simulink model "pumaModel"  (R2021b)
settings: Solver=VariableStepAuto  StartTime=0.0  StopTime=stopTime  FixedStep=.0001  RelTol=1e-3
values from neighbouring files (symbols this model uses):
  C = [0 c12_1*dq1 c13_1*dq3;c11_2*dq1 0 c22_2*dq2+c23_2*dq3;c11_3*dq1 c22_3*dq2 0]    [puma560ModifiedDynamics.m]
  dq_0 = [0 0 0]    [matlab.mat]
  fdControl = 2    [InitializationScript.m]
  fEE = 0    [InitializationScript.m]    (also in matlab.mat = 100)
  IC = [0;0;0]    [InitializationScript.m]    (also in matlab.mat = [0 0 0])
  m = 3    [matlab.mat]
  pathPoints = [IC,solution1,solution2,solution3,solution4,solution5,solution6]    [InitializationScript.m]    (also in matlab.mat = [0 0 0 4.71238898038 -1.57079632679 3.14159265359 3.14159265)
  q_0 = [0 0 0]    [matlab.mat]
  timePoints = [0 2 4 6 8 10 12]    [InitializationScript.m]    (also in matlab.mat = [0 2 4 6 8])
  velPoints = zeros(3,7)    [InitializationScript.m]    (also in matlab.mat = [0 0 0 0 0 0 0 0 0 0 0 0 ... (15 elements, 3x5)])
  X = [cos(q1)*(l2*cos(q2)+l3*sin(q2+q3));sin(q1)*(l2*cos(q2)+l3*sin(q2+q3));l1-l2*sin(q2)+l3*cos(q2+q3)]    [puma560ModifiedDynamics.m]
  Y = sym(zeros(3,size(cat(2,Y1,Y2,Y3),2)))    [puma560ModifiedDynamics.m]
undefined symbols (not defined in the file or in its folder): Z
libraries: sm_lib x96, nesl_utility x60, simulink x7, robotmaniplib x1, robotcorelib x1
(part 4 of 5)

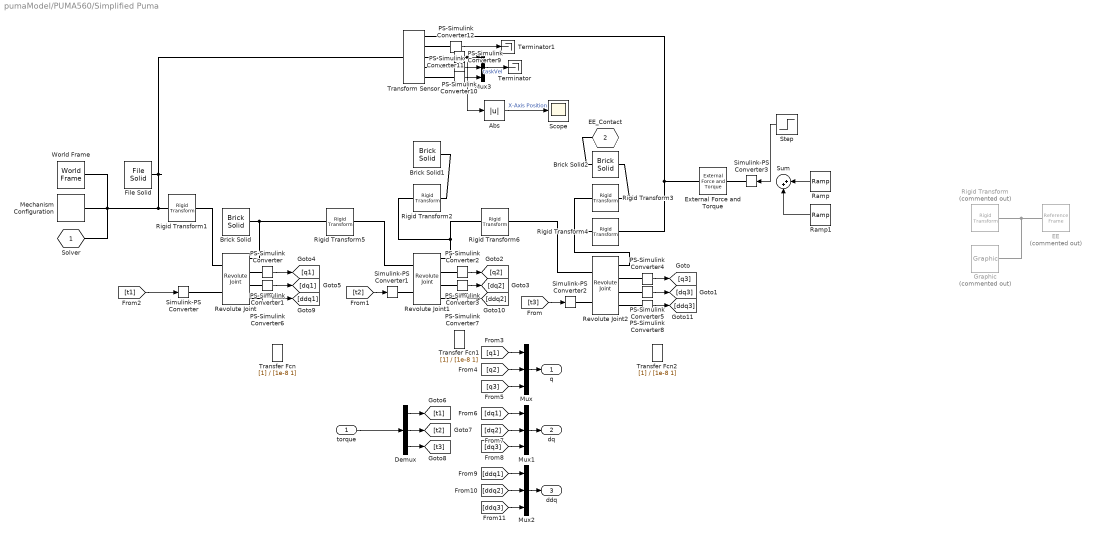
== system pumaModel/PUMA560/Simplified Puma ==
  torque : Inport
  Abs : Abs
  Brick Solid : sm_lib/Body Elements/Brick Solid  GraphicAmbientColor=[0.15 0.15 0.15 1.0]  BasedOnType=Density  BrickDimensions=[.1 .1 .1]  BrickDimensionUnits=m  CenterOfMass=[0 0 0]  CenterOfMassUnits=m  GraphicDiffuseColor=[1.0 0.0 0.2]  Density=1000  DensityUnits=kg/m^3  DoExposeReferenceFrame=on  GraphicEmissiveColor=[0.0 0.0 0.0 1.0]  ExportEntireGeometry=off  SerializedFrames=<Frames/>  MarkerShape=Sphere  MarkerSize=10  GraphicType=FromGeometry  InertiaType=PointMass  Mass=0  MassUnits=kg  MomentsOfInertia=[1 1 1]  MomentsOfInertiaUnits=kg*m^2  GraphicOpacity=1.0  ProductsOfInertia=[0 0 0]  ProductsOfInertiaUnits=kg*m^2  GraphicShininess=75  GraphicSpecularColor=[0.5 0.5 0.5 1.0]  GraphicVisPropType=SimpleVisualProperties
  Brick Solid1 : sm_lib/Body Elements/Brick Solid  GraphicAmbientColor=[0.15 0.15 0.15 1.0]  BasedOnType=Density  BrickDimensions=[.1 .1 .1]  BrickDimensionUnits=m  CenterOfMass=[0.216 0 0]  CenterOfMassUnits=m  GraphicDiffuseColor=[0.5 0.5 0.5]  Density=1000  DensityUnits=kg/m^3  DoExposeReferenceFrame=on  GraphicEmissiveColor=[0.0 0.0 0.0 1.0]  ExportEntireGeometry=off  SerializedFrames=<Frames/>  MarkerShape=Sphere  MarkerSize=10  GraphicType=FromGeometry  InertiaType=PointMass  Mass=15.46  MassUnits=kg  MomentsOfInertia=[0 0 15.46*.216]  MomentsOfInertiaUnits=kg*m^2  GraphicOpacity=1.0  ProductsOfInertia=[0 0 0]  ProductsOfInertiaUnits=kg*m^2  GraphicShininess=75  GraphicSpecularColor=[0.5 0.5 0.5 1.0]  GraphicVisPropType=SimpleVisualProperties
  Brick Solid2 : sm_lib/Body Elements/Brick Solid  GraphicAmbientColor=[0.15 0.15 0.15 1.0]  BasedOnType=Density  BrickDimensions=[.1 .1 .1]  BrickDimensionUnits=m  CenterOfMass=[0 0 0]  CenterOfMassUnits=m  GraphicDiffuseColor=[0.5 0.5 0.5]  Density=1000  DensityUnits=kg/m^3  DoExposeReferenceFrame=on  GraphicEmissiveColor=[0.0 0.0 0.0 1.0]  ExportEntireGeometry=on  SerializedFrames=<Frames/>  MarkerShape=Sphere  MarkerSize=10  GraphicType=FromGeometry  InertiaType=PointMass  Mass=9.55  MassUnits=kg  MomentsOfInertia=[1 1 1]  MomentsOfInertiaUnits=kg*m^2  GraphicOpacity=1.0  ProductsOfInertia=[0 0 0]  ProductsOfInertiaUnits=kg*m^2  GraphicShininess=75  GraphicSpecularColor=[0.5 0.5 0.5 1.0]  GraphicVisPropType=SimpleVisualProperties
  Demux : Demux  Outputs=3
  EE : sm_lib/Frames and Transforms/Reference Frame  Commented=on
  External Force and Torque : sm_lib/Forces and Torques/External Force and Torque  ForceResolutionFrame=World  EnableForceX=on  EnableForceY=off  EnableForceZ=off  EnableForce=off  TorqueResolutionFrame=AttachedFrame  EnableTorqueX=off  EnableTorqueY=off  EnableTorqueZ=off  EnableTorque=off
  File Solid : sm_lib/Body Elements/File Solid  ExtGeomFileName=.\Part1.STEP  UnitType=FromFile  ExtGeomFileUnits=m  StepReaderType=HEX  ExportConvexHullGeometry=off  InertiaType=Custom  Mass=1  MassUnits=kg  CenterOfMass=[0 0 0]  CenterOfMassUnits=m  MomentsOfInertia=[0 0 0]  MomentsOfInertiaUnits=kg*m^2  ProductsOfInertia=[0 0 0]  ProductsOfInertiaUnits=kg*m^2  BasedOnType=Density  Density=1000  DensityUnits=kg/m^3  DoExposeReferenceFrame=on  SerializedFrames=<Frames/>  GraphicType=FromGeometry  MarkerShape=Sphere  MarkerSize=10  GraphicVisPropType=SimpleVisualProperties  GraphicDiffuseColor=[0.5 0.5 0.5]  GraphicSpecularColor=[0.5 0.5 0.5 1.0]  GraphicAmbientColor=[0.15 0.15 0.15 1.0]  GraphicEmissiveColor=[0.0 0.0 0.0 1.0]  GraphicShininess=75  GraphicOpacity=1.0
  Graphic : sm_lib/Body Elements/Graphic  Commented=on  GraphicType=Marker  MarkerShape=Sphere  MarkerSize=10  GraphicVisPropType=SimpleVisualProperties  GraphicDiffuseColor=[1.0 0.0 0.2]  GraphicSpecularColor=[0.5 0.5 0.5 1.0]  GraphicAmbientColor=[0.15 0.15 0.15 1.0]  GraphicEmissiveColor=[0.0 0.0 0.0 1.0]  GraphicShininess=75  GraphicOpacity=1.0
  Mechanism Configuration : sm_lib/Utilities/Mechanism Configuration  UniformGravity=Constant  GravityVector=[0 0 -9.81]  GravityUnits=m/s^2  LinearizationDelta=0.001  JointModeTransitionNonlinearIterations=2
  Mux{,1..3} (4 alike) : Mux  Inputs=3
  PS-Simulink Converter{,1,9..12} (6 alike) : nesl_utility/PS-Simulink Converter  PhysicalDomain=network_engine_domain  SubClassName=ps_output  LeftPortType=input  RightPortType=output  PseudoPeriodic=off  Frequencies=[]  Unit=inherit  AffineConversion=off
      settings: SourceProductBaseCode=PW,SS
  PS-Simulink Converter2 : nesl_utility/PS-Simulink Converter  PhysicalDomain=network_engine_domain  SubClassName=ps_output  LeftPortType=input  RightPortType=output  PseudoPeriodic=off  Frequencies=[]  Unit=rad  AffineConversion=off
      settings: SourceProductBaseCode=PW,SS
  PS-Simulink Converter3 : nesl_utility/PS-Simulink Converter  PhysicalDomain=network_engine_domain  SubClassName=ps_output  LeftPortType=input  RightPortType=output  PseudoPeriodic=off  Frequencies=[]  Unit=rad/s  AffineConversion=off
      settings: SourceProductBaseCode=PW,SS
  PS-Simulink Converter4 : nesl_utility/PS-Simulink Converter  PhysicalDomain=network_engine_domain  SubClassName=ps_output  LeftPortType=input  RightPortType=output  PseudoPeriodic=off  Frequencies=[]  Unit=rad  AffineConversion=off
      settings: SourceProductBaseCode=PW,SS
  PS-Simulink Converter5 : nesl_utility/PS-Simulink Converter  PhysicalDomain=network_engine_domain  SubClassName=ps_output  LeftPortType=input  RightPortType=output  PseudoPeriodic=off  Frequencies=[]  Unit=rad/s  AffineConversion=off
      settings: SourceProductBaseCode=PW,SS
  PS-Simulink Converter6 : nesl_utility/PS-Simulink Converter  PhysicalDomain=network_engine_domain  SubClassName=ps_output  LeftPortType=input  RightPortType=output  PseudoPeriodic=off  Frequencies=[]  Unit=rad/s/s  AffineConversion=off
      settings: SourceProductBaseCode=PW,SS
  PS-Simulink Converter7 : nesl_utility/PS-Simulink Converter  PhysicalDomain=network_engine_domain  SubClassName=ps_output  LeftPortType=input  RightPortType=output  PseudoPeriodic=off  Frequencies=[]  Unit=rad/s/s  AffineConversion=off
      settings: SourceProductBaseCode=PW,SS
  PS-Simulink Converter8 : nesl_utility/PS-Simulink Converter  PhysicalDomain=network_engine_domain  SubClassName=ps_output  LeftPortType=input  RightPortType=output  PseudoPeriodic=off  Frequencies=[]  Unit=rad/s/s  AffineConversion=off
      settings: SourceProductBaseCode=PW,SS
  Ramp : simulink/Sources/Ramp  slope=-5  start=2  InitialOutput=0
  Ramp1 : simulink/Sources/Ramp  slope=5  start=6  InitialOutput=0
  Revolute Joint : sm_lib/Joints/Revolute Joint  JointMode=Normal  SenseConstraintForce=off  SenseConstraintForceX=off  SenseConstraintForceY=off  SenseConstraintForceZ=off  SenseConstraintTorque=off  SenseConstraintTorqueX=off  SenseConstraintTorqueY=off  SenseConstraintTorqueZ=off  SenseTotalForce=off  SenseTotalForceX=off  SenseTotalForceY=off  SenseTotalForceZ=off  SenseTotalTorque=off  SenseTotalTorqueX=off  SenseTotalTorqueY=off  SenseTotalTorqueZ=off  CompositeWrenchDir=FollowerOnBase  CompositeWrenchFrame=BaseFrame  EquilibriumPosition=0  EquilibriumPositionUnits=deg  SpringStiffness=0  SpringStiffnessUnits=N*m/deg  DampingCoefficient=0  DampingCoefficientUnits=N*m/(deg/s)  TorqueActuationMode=InputTorque  MotionActuationMode=ComputedMotion  SensePosition=on  SenseVelocity=on  SenseAcceleration=on  SenseTorqueForce=off  SenseLowerLimitTorqueForce=off  SenseUpperLimitTorqueForce=off  LowerLimitSpecify=off  LowerLimitBound=-90  LowerLimitBoundUnits=deg  LowerLimitStiffness=1e4  LowerLimitStiffnessUnits=N*m/deg  LowerLimitDamping=10  LowerLimitDampingUnits=N*m/(deg/s)  LowerLimitTransitionRegionWidth=0.1  LowerLimitTransitionRegionWidthUnits=deg  UpperLimitSpecify=off  UpperLimitBound=90  UpperLimitBoundUnits=deg  UpperLimitStiffness=1e4  UpperLimitStiffnessUnits=N*m/deg  UpperLimitDamping=10  UpperLimitDampingUnits=N*m/(deg/s)  UpperLimitTransitionRegionWidth=0.1  UpperLimitTransitionRegionWidthUnits=deg  PositionTargetSpecify=on  PositionTargetPriority=High  PositionTargetValue=IC(1)  PositionTargetValueUnits=rad  VelocityTargetSpecify=off  VelocityTargetPriority=High  VelocityTargetValue=0  VelocityTargetValueUnits=deg/s
  Revolute Joint1 : sm_lib/Joints/Revolute Joint  JointMode=Normal  SenseConstraintForce=off  SenseConstraintForceX=off  SenseConstraintForceY=off  SenseConstraintForceZ=off  SenseConstraintTorque=off  SenseConstraintTorqueX=off  SenseConstraintTorqueY=off  SenseConstraintTorqueZ=off  SenseTotalForce=off  SenseTotalForceX=off  SenseTotalForceY=off  SenseTotalForceZ=off  SenseTotalTorque=off  SenseTotalTorqueX=off  SenseTotalTorqueY=off  SenseTotalTorqueZ=off  CompositeWrenchDir=FollowerOnBase  CompositeWrenchFrame=BaseFrame  EquilibriumPosition=0  EquilibriumPositionUnits=deg  SpringStiffness=0  SpringStiffnessUnits=N*m/deg  DampingCoefficient=0  DampingCoefficientUnits=N*m/(deg/s)  TorqueActuationMode=InputTorque  MotionActuationMode=ComputedMotion  SensePosition=on  SenseVelocity=on  SenseAcceleration=on  SenseTorqueForce=off  SenseLowerLimitTorqueForce=off  SenseUpperLimitTorqueForce=off  LowerLimitSpecify=off  LowerLimitBound=-90  LowerLimitBoundUnits=deg  LowerLimitStiffness=1e4  LowerLimitStiffnessUnits=N*m/deg  LowerLimitDamping=10  LowerLimitDampingUnits=N*m/(deg/s)  LowerLimitTransitionRegionWidth=0.1  LowerLimitTransitionRegionWidthUnits=deg  UpperLimitSpecify=off  UpperLimitBound=90  UpperLimitBoundUnits=deg  UpperLimitStiffness=1e4  UpperLimitStiffnessUnits=N*m/deg  UpperLimitDamping=10  UpperLimitDampingUnits=N*m/(deg/s)  UpperLimitTransitionRegionWidth=0.1  UpperLimitTransitionRegionWidthUnits=deg  PositionTargetSpecify=on  PositionTargetPriority=High  PositionTargetValue=IC(2)  PositionTargetValueUnits=rad  VelocityTargetSpecify=off  VelocityTargetPriority=High  VelocityTargetValue=0  VelocityTargetValueUnits=deg/s
  Revolute Joint2 : sm_lib/Joints/Revolute Joint  JointMode=Normal  SenseConstraintForce=off  SenseConstraintForceX=off  SenseConstraintForceY=off  SenseConstraintForceZ=off  SenseConstraintTorque=off  SenseConstraintTorqueX=off  SenseConstraintTorqueY=off  SenseConstraintTorqueZ=off  SenseTotalForce=off  SenseTotalForceX=off  SenseTotalForceY=off  SenseTotalForceZ=off  SenseTotalTorque=off  SenseTotalTorqueX=off  SenseTotalTorqueY=off  SenseTotalTorqueZ=off  CompositeWrenchDir=FollowerOnBase  CompositeWrenchFrame=BaseFrame  EquilibriumPosition=0  EquilibriumPositionUnits=deg  SpringStiffness=0  SpringStiffnessUnits=N*m/deg  DampingCoefficient=0  DampingCoefficientUnits=N*m/(deg/s)  TorqueActuationMode=InputTorque  MotionActuationMode=ComputedMotion  SensePosition=on  SenseVelocity=on  SenseAcceleration=on  SenseTorqueForce=off  SenseLowerLimitTorqueForce=off  SenseUpperLimitTorqueForce=off  LowerLimitSpecify=off  LowerLimitBound=-90  LowerLimitBoundUnits=deg  LowerLimitStiffness=1e4  LowerLimitStiffnessUnits=N*m/deg  LowerLimitDamping=10  LowerLimitDampingUnits=N*m/(deg/s)  LowerLimitTransitionRegionWidth=0.1  LowerLimitTransitionRegionWidthUnits=deg  UpperLimitSpecify=off  UpperLimitBound=90  UpperLimitBoundUnits=deg  UpperLimitStiffness=1e4  UpperLimitStiffnessUnits=N*m/deg  UpperLimitDamping=10  UpperLimitDampingUnits=N*m/(deg/s)  UpperLimitTransitionRegionWidth=0.1  UpperLimitTransitionRegionWidthUnits=deg  PositionTargetSpecify=on  PositionTargetPriority=High  PositionTargetValue=IC(3)  PositionTargetValueUnits=rad  VelocityTargetSpecify=off  VelocityTargetPriority=High  VelocityTargetValue=0  VelocityTargetValueUnits=deg/s
  Rigid Transform : sm_lib/Frames and Transforms/Rigid Transform  Commented=on  TranslationMethod=StandardAxis  TranslationStandardOffset=.08029876  TranslationLengthUnit=m  TranslationStandardAxis=+Z  TranslationCartesianOffset=[0 0 0]  TranslationROffset=0  TranslationROffsetUnits=m  TranslationZOffset=0  TranslationZOffsetUnits=m  TranslationThetaOffset=0  TranslationThetaOffsetUnits=deg  RotationMethod=None  RotationAngleUnits=deg  RotationStandardAxis=+Z  RotationAngle=0.0  RotationArbitraryAxis=[0 0 1]  FollAlignAxisA=+X  BaseAlignAxisA=+Y  FollAlignAxisB=+Y  BaseAlignAxisB=+Z  RotationSequenceAxes=FollowerAxes  RotationSequence=XYX  RotationSequenceAngles=[0 0 0]  RotationSequenceAnglesUnits=deg  RotationMatrix=[1 0 0; 0 1 0; 0 0 1]
  Rigid Transform1 : sm_lib/Frames and Transforms/Rigid Transform  TranslationMethod=Cartesian  TranslationStandardOffset=0  TranslationLengthUnit=m  TranslationStandardAxis=+Z  TranslationCartesianOffset=[0 0 0.6731]  TranslationROffset=0  TranslationROffsetUnits=m  TranslationZOffset=0  TranslationZOffsetUnits=m  TranslationThetaOffset=0  TranslationThetaOffsetUnits=deg  RotationMethod=RotationMatrix  RotationAngleUnits=deg  RotationStandardAxis=+X  RotationAngle=90  RotationArbitraryAxis=[0 0 1]  FollAlignAxisA=+X  BaseAlignAxisA=+Y  FollAlignAxisB=+Y  BaseAlignAxisB=+Z  RotationSequenceAxes=FollowerAxes  RotationSequence=XYX  RotationSequenceAngles=[0 0 0]  RotationSequenceAnglesUnits=deg  RotationMatrix=eye(3)
  Rigid Transform2 : sm_lib/Frames and Transforms/Rigid Transform  TranslationMethod=Cartesian  TranslationStandardOffset=0  TranslationLengthUnit=m  TranslationStandardAxis=+Z  TranslationCartesianOffset=[.216 0 0]  TranslationROffset=0  TranslationROffsetUnits=m  TranslationZOffset=0  TranslationZOffsetUnits=m  TranslationThetaOffset=0  TranslationThetaOffsetUnits=deg  RotationMethod=RotationMatrix  RotationAngleUnits=deg  RotationStandardAxis=+X  RotationAngle=90  RotationArbitraryAxis=[0 0 1]  FollAlignAxisA=+X  BaseAlignAxisA=+Y  FollAlignAxisB=+Y  BaseAlignAxisB=+Z  RotationSequenceAxes=FollowerAxes  RotationSequence=XYX  RotationSequenceAngles=[0 0 0]  RotationSequenceAnglesUnits=deg  RotationMatrix=eye(3)
  Rigid Transform3 : sm_lib/Frames and Transforms/Rigid Transform  TranslationMethod=Cartesian  TranslationStandardOffset=0  TranslationLengthUnit=m  TranslationStandardAxis=+Z  TranslationCartesianOffset=[0 -0.164 0]  TranslationROffset=0  TranslationROffsetUnits=m  TranslationZOffset=0  TranslationZOffsetUnits=m  TranslationThetaOffset=0  TranslationThetaOffsetUnits=deg  RotationMethod=None  RotationAngleUnits=deg  RotationStandardAxis=+X  RotationAngle=90  RotationArbitraryAxis=[0 0 1]  FollAlignAxisA=+X  BaseAlignAxisA=+Y  FollAlignAxisB=+Y  BaseAlignAxisB=+Z  RotationSequenceAxes=FollowerAxes  RotationSequence=XYX  RotationSequenceAngles=[0 0 0]  RotationSequenceAnglesUnits=deg  RotationMatrix=[1 0 0;0 0 -1;0 1 0]
  Rigid Transform4 : sm_lib/Frames and Transforms/Rigid Transform  TranslationMethod=Cartesian  TranslationStandardOffset=0  TranslationLengthUnit=m  TranslationStandardAxis=+Z  TranslationCartesianOffset=[0 -0.434 0]  TranslationROffset=0  TranslationROffsetUnits=m  TranslationZOffset=0  TranslationZOffsetUnits=m  TranslationThetaOffset=0  TranslationThetaOffsetUnits=deg  RotationMethod=None  RotationAngleUnits=deg  RotationStandardAxis=+X  RotationAngle=90  RotationArbitraryAxis=[0 0 1]  FollAlignAxisA=+X  BaseAlignAxisA=+Y  FollAlignAxisB=+Y  BaseAlignAxisB=+Z  RotationSequenceAxes=FollowerAxes  RotationSequence=XYX  RotationSequenceAngles=[0 0 0]  RotationSequenceAnglesUnits=deg  RotationMatrix=[1 0 0;0 0 -1;0 1 0]
  Rigid Transform5 : sm_lib/Frames and Transforms/Rigid Transform  TranslationMethod=None  TranslationStandardOffset=0  TranslationLengthUnit=m  TranslationStandardAxis=+Z  TranslationCartesianOffset=[0 0 0]  TranslationROffset=0  TranslationROffsetUnits=m  TranslationZOffset=0  TranslationZOffsetUnits=m  TranslationThetaOffset=0  TranslationThetaOffsetUnits=deg  RotationMethod=RotationMatrix  RotationAngleUnits=deg  RotationStandardAxis=+X  RotationAngle=90  RotationArbitraryAxis=[0 0 1]  FollAlignAxisA=+X  BaseAlignAxisA=+Y  FollAlignAxisB=+Y  BaseAlignAxisB=+Z  RotationSequenceAxes=FollowerAxes  RotationSequence=XYX  RotationSequenceAngles=[0 0 0]  RotationSequenceAnglesUnits=deg  RotationMatrix=[1 0 0;0 0 1;0 -1 0]
  Rigid Transform6 : sm_lib/Frames and Transforms/Rigid Transform  TranslationMethod=Cartesian  TranslationStandardOffset=0  TranslationLengthUnit=m  TranslationStandardAxis=+Z  TranslationCartesianOffset=[.432 0 0]  TranslationROffset=0  TranslationROffsetUnits=m  TranslationZOffset=0  TranslationZOffsetUnits=m  TranslationThetaOffset=0  TranslationThetaOffsetUnits=deg  RotationMethod=RotationMatrix  RotationAngleUnits=deg  RotationStandardAxis=+X  RotationAngle=90  RotationArbitraryAxis=[0 0 1]  FollAlignAxisA=+X  BaseAlignAxisA=+Y  FollAlignAxisB=+Y  BaseAlignAxisB=+Z  RotationSequenceAxes=FollowerAxes  RotationSequence=XYX  RotationSequenceAngles=[0 0 0]  RotationSequenceAnglesUnits=deg  RotationMatrix=eye(3)
  Scope : Scope
  Simulink-PS Converter : nesl_utility/Simulink-PS Converter  PhysicalDomain=network_engine_domain  SubClassName=ps_input  LeftPortType=input  RightPortType=output  PseudoPeriodic=off  Frequencies=[]  NoiseDistribution=none  NoiseParameters=[]  Unit=N*m  AffineConversion=off  FilteringAndDerivatives=provide  SimscapeFilterOrder=1  InputFilterTimeConstant=0.001  UdotUserProvided=0
      settings: SourceProductBaseCode=PW,SS
  Simulink-PS Converter1 : nesl_utility/Simulink-PS Converter  PhysicalDomain=network_engine_domain  SubClassName=ps_input  LeftPortType=input  RightPortType=output  PseudoPeriodic=off  Frequencies=[]  NoiseDistribution=none  NoiseParameters=[]  Unit=N*m  AffineConversion=off  FilteringAndDerivatives=provide  SimscapeFilterOrder=1  InputFilterTimeConstant=0.001  UdotUserProvided=0
      settings: SourceProductBaseCode=PW,SS
  Simulink-PS Converter2 : nesl_utility/Simulink-PS Converter  PhysicalDomain=network_engine_domain  SubClassName=ps_input  LeftPortType=input  RightPortType=output  PseudoPeriodic=off  Frequencies=[]  NoiseDistribution=none  NoiseParameters=[]  Unit=N*m  AffineConversion=off  FilteringAndDerivatives=provide  SimscapeFilterOrder=1  InputFilterTimeConstant=0.001  UdotUserProvided=0
      settings: SourceProductBaseCode=PW,SS
  Simulink-PS Converter3 : nesl_utility/Simulink-PS Converter  PhysicalDomain=network_engine_domain  SubClassName=ps_input  LeftPortType=input  RightPortType=output  PseudoPeriodic=off  Frequencies=[]  NoiseDistribution=none  NoiseParameters=[]  Unit=1  AffineConversion=off  FilteringAndDerivatives=provide  SimscapeFilterOrder=1  InputFilterTimeConstant=0.001  UdotUserProvided=0
      settings: SourceProductBaseCode=PW,SS
  Step : Step  After=-20  SampleTime=0
  Sum : Sum  Inputs=|++
  Terminator : Terminator
  Terminator1 : Terminator
  Transfer Fcn : TransferFcn  Denominator=[1e-8 1]
  Transfer Fcn1 : TransferFcn  Denominator=[1e-8 1]
  Transfer Fcn2 : TransferFcn  Denominator=[1e-8 1]
  Transform Sensor : sm_lib/Frames and Transforms/Transform Sensor  MeasurementFrame=Base  SenseAngle=off  SenseAxis=off  SenseAngle1=off  SenseAngle2=off  SenseAngle3=off  SenseQ=off  SenseR=on  SenseOmegaX=off  SenseOmegaY=off  SenseOmegaZ=off  SenseOmega1=off  SenseOmega2=off  SenseOmega3=off  SenseQDot=off  SenseRDot=off  SenseAlphaX=off  SenseAlphaY=off  SenseAlphaZ=off  SenseAlpha1=off  SenseAlpha2=off  SenseAlpha3=off  SenseQDDot=off  SenseRDDot=off  SenseX=on  SenseY=on  SenseZ=on  SenseRad=off  SenseAzim=off  SenseDist=off  SenseInc=off  SenseXDot=off  SenseYDot=off  SenseZDot=off  SenseRadDot=off  SenseAzimDot=off  SenseDistDot=off  SenseIncDot=off  SenseXDDot=off  SenseYDDot=off  SenseZDDot=off  SenseRadDDot=off  SenseAzimDDot=off  SenseDistDDot=off  SenseIncDDot=off
  World Frame : sm_lib/Frames and Transforms/World Frame
  Solver : PMIOPort  Tag=PMCPort  Side=Left
  EE_Contact : PMIOPort  Tag=PMCPort  Port=2  Side=Right
  q : Outport
  dq : Outport  Port=2
  ddq : Outport  Port=3
  wires:
  [t1] -> Simulink-PS Converter/1
  Mux2/1 -> ddq/1
  [ddq3] -> Mux2/3
  [ddq1] -> Mux2/1
  [ddq2] -> Mux2/2
  Mux/1 -> q/1
  [dq2] -> Mux1/2
  [q3] -> Mux/3
  [dq1] -> Mux1/1
  PS-Simulink Converter1/1 -> [dq1]
  PS-Simulink Converter4/1 -> [q3]
  PS-Simulink Converter2/1 -> [q2]
  Demux/1 -> [t1]
  Demux/3 -> [t3]
  PS-Simulink Converter/1 -> [q1]
  [dq3] -> Mux1/3
  Mux1/1 -> dq/1
  [q1] -> Mux/1
  [t3] -> Simulink-PS Converter2/1
  PS-Simulink Converter5/1 -> [dq3]
  PS-Simulink Converter3/1 -> [dq2]
  Demux/2 -> [t2]
  [q2] -> Mux/2
  [t2] -> Simulink-PS Converter1/1
  torque/1 -> Demux/1
  PS-Simulink Converter6/1 -> [ddq1]
  PS-Simulink Converter7/1 -> [ddq2]
  PS-Simulink Converter8/1 -> [ddq3]
  PS-Simulink Converter12/1 -> Terminator1/1
  Mux3/1 -> Terminator/1  "taskVel"
  PS-Simulink Converter10/1 -> Mux3/2
  PS-Simulink Converter11/1 -> Mux3/3
  PS-Simulink Converter9/1 -> Abs/1, Mux3/1
  Abs/1 -> Scope/1  "X-Axis Position"
  Ramp/1 -> Sum/1
  Ramp1/1 -> Sum/2
  Step/1 -> Simulink-PS Converter3/1
  connections:
  Revolute Joint2/RConn4 -- PS-Simulink Converter8/LConn1
  PS-Simulink Converter7/LConn1 -- Revolute Joint1/RConn4
  Revolute Joint/RConn4 -- PS-Simulink Converter6/LConn1
  Graphic/RConn1 -- EE/RConn1 -- Rigid Transform/RConn1
  Simulink-PS Converter2/RConn1 -- Revolute Joint2/LConn2
  Revolute Joint/RConn3 -- PS-Simulink Converter1/LConn1
  PS-Simulink Converter/LConn1 -- Revolute Joint/RConn2
  Revolute Joint2/RConn3 -- PS-Simulink Converter5/LConn1
  Simulink-PS Converter1/RConn1 -- Revolute Joint1/LConn2
  Simulink-PS Converter/RConn1 -- Revolute Joint/LConn2
  Rigid Transform5/RConn1 -- Revolute Joint1/LConn1
  Revolute Joint1/RConn3 -- PS-Simulink Converter3/LConn1
  Rigid Transform3/LConn1 -- Rigid Transform4/LConn1 -- Revolute Joint2/RConn1
  Rigid Transform6/LConn1 -- Rigid Transform2/LConn1 -- Revolute Joint1/RConn1
  Revolute Joint2/LConn1 -- Rigid Transform6/RConn1
  Rigid Transform5/LConn1 -- Brick Solid/RConn1 -- Revolute Joint/RConn1
  PS-Simulink Converter4/LConn1 -- Revolute Joint2/RConn2
  Revolute Joint1/RConn2 -- PS-Simulink Converter2/LConn1
  Revolute Joint/LConn1 -- Rigid Transform1/RConn1
  Rigid Transform1/LConn1 -- Transform Sensor/LConn1 -- File Solid/RConn1 -- Solver/RConn1 -- Mechanism Configuration/RConn1 -- World Frame/RConn1
  Brick Solid1/RConn1 -- Rigid Transform2/RConn1
  Rigid Transform3/RConn1 -- Brick Solid2/RConn1
  EE_Contact/RConn1 -- Brick Solid2/LConn1
  Simulink-PS Converter3/RConn1 -- External Force and Torque/LConn1
  External Force and Torque/RConn1 -- Transform Sensor/RConn1 -- Rigid Transform4/RConn1
  Transform Sensor/RConn5 -- PS-Simulink Converter11/LConn1
  Transform Sensor/RConn3 -- PS-Simulink Converter9/LConn1
  PS-Simulink Converter12/LConn1 -- Transform Sensor/RConn2
  Transform Sensor/RConn4 -- PS-Simulink Converter10/LConn1

== system pumaModel/Controller/PD + Gravity Compensation/PD + Gravity Compensation ==
  qd : Inport
  dq : Inport  Port=2
  q : Inport  Port=3
  Demux : Demux  Outputs=3
  Demux1 : Demux  Outputs=3
  Gain : Gain  Gain=[50 0 0;0 50 0;0 0 50]  Multiplication=Matrix(K*u) (u vector)
  Gain1 : Gain  Gain=-[20 0 0;0 20 0;0 0 15]  Multiplication=Matrix(K*u) (u vector)
  Gravity Torque : robotmaniplib/Gravity Torque  RigidBodyTree=PUMA560  SimulateUsing=Interpreted execution
  MATLAB Function : MATLAB Function  TreatAsAtomicUnit=on
  Mux : Mux  Inputs=3
  Scope : Scope  NumInputPorts=2
  Sum : Sum  Inputs=-+|
  Sum1 : Sum  Inputs=-+|
  Sum2 : Sum  Inputs=||+++
  Sum3 : Sum  Inputs=-+|
  torque : Outport
  wires:
  Sum3/1 -> Mux/3
  Mux/1 -> Gain/1
  dq/1 -> Gain1/1
  Demux/1 -> Sum/1
  Sum2/1 -> torque/1
  Demux/2 -> Sum1/1
  q/1 -> Gravity Torque/1, Demux/1, MATLAB Function/1(q)
  Sum1/1 -> Mux/2
  Sum/1 -> Mux/1
  Demux/3 -> Sum3/1
  Demux1/2 -> Sum1/2
  Demux1/3 -> Sum3/2
  Demux1/1 -> Sum/2
  qd/1 -> Demux1/1
  MATLAB Function/1(gTorque) -> Scope/2, Sum2/1
  Gain/1 -> Sum2/2
  Gain1/1 -> Sum2/3
  Gravity Torque/1 -> Scope/1

== system pumaModel/Controller/Parrelel Force and Motion Control/Force Control ==
  F : Inport
  Fd : Inport  Port=2
  1/Ka : Gain  Gain=1/20
  Integrator : Integrator
  Integrator1 : Integrator
  Kv : Gain  Gain=95
  Scope1 : Scope  NumInputPorts=3
  Selector : Selector  InputPortWidth=3  IndexOptions=Starting index (dialog)  Indices=[1]  OutputSizes=1
  Selector1 : Selector  InputPortWidth=3  IndexOptions=Starting index (dialog)  Indices=[1]  OutputSizes=1
  Selector2 : Selector  InputPortWidth=3  IndexOptions=Starting index (dialog)  Indices=[1]  OutputSizes=1
  Sum : Sum  Inputs=|+-
  Sum1 : Sum  Inputs=|+-
  pf : Outport
  pfDot : Outport  Port=2
  pfDotDot : Outport  Port=3
  wires:
  Integrator/1 -> Integrator1/1, Selector1/1, pfDot/1, Kv/1
  Integrator1/1 -> Selector/1, pf/1
  Kv/1 -> Sum/2
  Sum/1 -> 1/Ka/1
  Sum1/1 -> Sum/1
  F/1 -> Sum1/2
  Fd/1 -> Sum1/1
  1/Ka/1 -> Selector2/1, pfDotDot/1, Integrator/1
  Selector/1 -> Scope1/1
  Selector1/1 -> Scope1/2
  Selector2/1 -> Scope1/3

== matlab function pumaModel/Controller/Impedance No Measurements/TaskSpaceImpedance_NoMeasurements ==
  data: q input; dq input; ddq input; qd input; dqd input; torque output; ddqd input; previousJacIn input; previousJacOut output; Hp output
function [torque,previousJacOut,Hp]    = ImpedanceControllerTaskSpace_Lectures_NoForceMeasurements(q,dq,ddq,qd,dqd,ddqd,previousJacIn)
%% Joint Space variables
q1 = q(1);
q2 = q(2);
q3 = q(3);

dq1 = dq(1);
dq2 = dq(2);
dq3 = dq(3);

qd1 = qd(1);
qd2 = qd(2);
qd3 = qd(3);

% dqd1 = dqd(1);
% dqd2 = dqd(2);
% dqd3 = dqd(3);

%% Manipulator Geometry
l1 = 0.6731;
l2 = 0.432;
l3 = 0.434;
lc2 = 0.216;
lc3 = 0.164;
m2 = 15.46;
m3 = 9.55;
J = 0.302;

J1 = m3 * lc3^2;
J12 = (m2 * lc2^2) + (m3 * l2^2);
J13 = l2 * lc3 * m3;


h11 = J + J1 * (sin(q2 + q3))^2 + J12 * (cos(q2))^2 + 2 * J13 * cos(q2) * sin(q2+q3);
h22 = J1 + J12 + 2 * J13 * sin(q3);
h23 = J1 + J13 * sin(q3);
h32 = h23;
h33 = J1;

H = [h11, 0 ,0 ;
    0 , h22, h23;
    0 , h32, h33];

c12_1 = J1 * sin(2 * (q1 + q2)) - J12 * sin(2 * q2) + 2 * J13 * cos(2 * q2 +q3);
c13_1 = J1 * sin(2 * (q2 + q3)) + 2 * J13 * cos(q2) * cos(q2 + q3);
c11_2 = (1/2) * (-J1 * sin(2 * (q2 + q3)) + J12 * sin(2 * q2) - 2 * J13 * cos(2 * q2 + q3));
c22_2 = 2 * J13 * cos(q3);
c23_2 = J13 * cos(q3);
c22_3 = -J13 * cos(q3)* dq2;%NEED TO CHECK IF THIS IS CORRECT
c11_3 = (-1/2) * (J1 * sin(2 * (q2 + q3)) + J13 * cos(q2) * cos(q2 + q3));

C = [0, c12_1 * dq1, c13_1 * dq3;
    c11_2 * dq1, 0 , (c22_2)* dq2 + (c23_2)*dq3;
    c11_3 * dq1, c22_3 * dq2, 0];

g = 9.81;

g21 = -g * (lc3 * m3 * sin(q2 + q3) + lc2 * m2 * cos(q2) + l2 * m3 * cos(q2));
g31 = -g * (lc3 * m3 * sin(q2 + q3));

G = [0;
    g21;
    g31];

%% Define the Jacobian
jac=[-sin(q1)*(l3*sin(q2 + q3) + l2*cos(q2)), cos(q1)*(l3*cos(q2 + q3) - l2*sin(q2)), l3*cos(q2 + q3)*cos(q1);
 cos(q1)*(l3*sin(q2 + q3) + l2*cos(q2)), sin(q1)*(l3*cos(q2 + q3) - l2*sin(q2)), l3*cos(q2 + q3)*sin(q1);
                                      0,         - l3*sin(q2 + q3) - l2*cos(q2),        -l3*sin(q2 + q3)];
                                  
%% Define the derivative of the jacobian
dJac=[- sin(q1)*(l3*cos(q2 + q3)*(dq2 + dq3) - l2*sin(q2)*dq2) - cos(q1)*(l2*cos(q2) + l3*sin(q2 + q3))*dq1,   sin(q1)*dq1*(l2*sin(q2) - l3*cos(q2 + q3)) - cos(q1)*(l3*sin(q2 + q3)*(dq2 + dq3) + l2*cos(q2)*dq2), - l3*sin(q1)*cos(q2 + q3)*dq1 - l3*cos(q1)*sin(q2 + q3)*(dq2 + dq3);
  cos(q1)*(l3*cos(q2 + q3)*(dq2 + dq3) - l2*sin(q2)*dq2) - sin(q1)*(l2*cos(q2) + l3*sin(q2 + q3))*dq1, - sin(q1)*(l3*sin(q2 + q3)*(dq2 + dq3) + l2*cos(q2)*dq2) - cos(q1)*(l2*sin(q2) - l3*cos(q2 + q3))*dq1,   l3*cos(q1)*cos(q2 + q3)*dq1 - l3*sin(q1)*sin(q2 + q3)*(dq2 + dq3);
                                                                                                                                                                        0,                                                                                    l2*sin(q2)*dq2 - l3*cos(q2 + q3)*(dq2 + dq3),                                                               -l3*cos(q2 + q3)*(dq2 + dq3)];

%% Define the task space matrices
%Check to make sure we haven't hit a singularity
if det(jac)<10e-4
    jac=previousJacIn;
    previousJacOut=previousJacIn;
else
    previousJacOut=jac;
end

Hp=inv(transpose(jac))*H*inv(jac);
Cp=inv(transpose(jac))*C*inv(jac)-Hp*dJac*inv(jac);
Gp=inv(transpose(jac))*G;

%% Equivalent Task Space Vectors
p=[cos(q1)*(l3*sin(q2 + q3) + l2*cos(q2));sin(q1)*(l3*sin(q2 + q3) + l2*cos(q2));l1 + l3*cos(q2 + q3) - l2*sin(q2)];
pd=[cos(qd1)*(l3*sin(qd2 + qd3) + l2*cos(qd2));sin(qd1)*(l3*sin(qd2 + qd3) + l2*cos(qd2));l1 + l3*cos(qd2 + qd3) - l2*sin(qd2)];

dp=jac*dq;
dpd=jac*dqd;

ddpd=jac*ddqd+dJac*dqd;

                                  

%% Function output
%Define the stiffness and damping matrix below for task space directions
Km=[100 0 0;0 15000 0;0 0 15000];
Dm=[50 0 0;0 50 0;0 0 50];

jacT=transpose(jac);
torque=jacT*(Hp*ddpd+Dm*(dpd-dp)+Km*(pd-p)+Cp*dp+Gp);
% torque=G;
test=det(jac);

== matlab function pumaModel/Controller/Robust Control/RobustControl ==
  data: q input; dq input; qd input; dqd input; u output; ddqd input
function u  = ImpedanceControllerTaskSpace(q,dq,qd,dqd,ddqd)
%Unpackage the incoming reference/measured states
q1 = q(1);
q2 = q(2);
q3 = q(3);

qd1 = qd(1);
qd2 = qd(2);
qd3 = qd(3);

dq1 = dq(1);
dq2 = dq(2);
dq3 = dq(3);

dqd1 = dqd(1);
dqd2 = dqd(2);
dqd3 = dqd(3);

ddqd1=ddqd(1);
ddqd2=ddqd(2);
ddqd3=ddqd(3);

%Define parameters
kd1=20;
kd2=20;
kd3=20;

kp1=50;
kp2=50;
kp3=50;

%Define all our own variables
qError=q-qd;
dqError=dq-dqd;

%Define State equation vectors/matrices
x=[qError;dqError];

B=[0     0     0;
     0     0     0;
     0     0     0;
     1     0     0;
     0     1     0;
     0     0     1];

 P=[0.1253         0         0   -0.5000         0         0;
         0    0.1253         0         0   -0.5000         0;
         0         0    0.1253         0         0   -0.5000;
   -0.5000         0         0    2.5250         0         0;
         0   -0.5000         0         0    2.5250         0;
         0         0   -0.5000         0         0    2.5250];

%Define our beta function
beta=(4*(kd1*(dq1 - dqd1) - ddqd1 + kp1*(q1 - qd1))^2 + 4*(kd2*(dq2 - dqd2) - ddqd2 + kp2*(q2 - qd2))^2 + 3*(kd3*(dq3 - dqd3) - ddqd3 + kp3*(q3 - qd3))^2 + 5*dq1^4 + 3*dq3^4 + dq2^6 + 4*dq1^2*dq2^2 + dq2^2*dq3^2 + 3)^(1/2);

%Define our maximum parameter error (thetaStar)
% thetaStar=.00529;%This is the norm of the thetaTilda vector if we were to calculate it
thetaStar=100;

%Define Y
Y=[-cos(q2)^2*(kd1*(dq1 - dqd1) - ddqd1 + kp1*(q1 - qd1)), -sin(q2 + q3)*cos(q2)*(kd1*(dq1 - dqd1) - ddqd1 + kp1*(q1 - qd1)), -sin(q2 + q3)^2*(kd1*(dq1 - dqd1) - ddqd1 + kp1*(q1 - qd1)), ddqd1 - kd1*(dq1 - dqd1) - kp1*(q1 - qd1), dq1*dq2*sin(2*q1 + 2*q2), dq1*dq2*cos(2*q2 + q3), dq1*dq2*sin(2*q2), dq1*dq2, dq3^2*cos(q2 + q3)*cos(q2), dq3^2*sin(2*q2 + 2*q3),                                                    0,                                         0,                                                    0,                                         0,                      0,                    0,               0,               0,             0,       0,            0,                                                    0,                                         0,                                         0,                          0,                      0,             0,            0;
                                                     0,                                                                 0,                                                           0,                                         0,                        0,                      0,                 0,       0,                          0,                      0, -sin(q3)*(kd2*(dq2 - dqd2) - ddqd2 + kp2*(q2 - qd2)), ddqd2 - kd2*(dq2 - dqd2) - kp2*(q2 - qd2), -sin(q3)*(kd3*(dq3 - dqd3) - ddqd3 + kp3*(q3 - qd3)), ddqd3 - kd3*(dq3 - dqd3) - kp3*(q3 - qd3), dq1^2*sin(2*q2 + 2*q3), dq1^2*cos(2*q2 + q3), dq1^2*sin(2*q2), dq2*dq3*cos(q3), dq3^2*cos(q3), cos(q2), sin(q2 + q3),                                                    0,                                         0,                                         0,                          0,                      0,             0,            0;
                                                     0,                                                                 0,                                                           0,                                         0,                        0,                      0,                 0,       0,                          0,                      0,                                                    0,                                         0,                                                    0,                                         0,                      0,                    0,               0,               0,             0,       0,            0, -sin(q3)*(kd2*(dq2 - dqd2) - ddqd2 + kp2*(q2 - qd2)), ddqd2 - kd2*(dq2 - dqd2) - kp2*(q2 - qd2), ddqd3 - kd3*(dq3 - dqd3) - kp3*(q3 - qd3), dq1^2*cos(q2 + q3)*cos(q2), dq1^2*sin(2*q2 + 2*q3), dq2^3*cos(q3), sin(q2 + q3)];
%Define theta0
theta0=transpose([2.5, 1.35, 0.257, 0.302, 0.257, 1.35, -1.0, -2.5, 1.35, 0.257, 1.35, 2.76, 0.677, 0.257, -0.128, -1.35, 2.5, 1.35, 0.677, -73.2, -15.4, 0.677, 0.257, 0.257, -0.338, -0.128, -0.677, -15.4]);

%Define etta
E=0.05;%May need to change this value later, this was assigned arbitrairly 

%Define max and min eigen values
lambdaMax=23.3585;
lambdaMin=0.2265;

%Define our robust term (u0)
u0=-lambdaMax/(E*lambdaMin)*(beta*thetaStar)^2*transpose(B)*P*x;

%Define our complete control law
u=Y*theta0+u0;
test=beta*thetaStar*norm(transpose(B)*P*x);

== matlab function pumaModel/Controller/Parrelel Force and Motion Control/Parrellel Decompostion+Tracking Control+ID ==
  data: q input; dq input; qd input; dqd input; ddqd input; pf input; dpf input; ddpf input; torque output; f input; previousJacOut output; previousJacIn input; test output
function [torque,previousJacOut,test]     = ImpedanceControllerTaskSpace_Lectures_NoForceMeasurements(q,dq,qd,dqd,ddqd,pf,dpf,ddpf,f,previousJacIn)
%% Joint Space variables
q1 = q(1);
q2 = q(2);
q3 = q(3);

dq1 = dq(1);
dq2 = dq(2);
dq3 = dq(3);

qd1 = qd(1);
qd2 = qd(2);
qd3 = qd(3);

%% Manipulator Geometry
l1 = 0.6731;
l2 = 0.432;
l3 = 0.434;
lc2 = 0.216;
lc3 = 0.164;
m2 = 15.46;
m3 = 9.55;
J = 0.302;

J1 = m3 * lc3^2;
J12 = (m2 * lc2^2) + (m3 * l2^2);
J13 = l2 * lc3 * m3;


h11 = J + J1 * (sin(q2 + q3))^2 + J12 * (cos(q2))^2 + 2 * J13 * cos(q2) * sin(q2+q3);
h22 = J1 + J12 + 2 * J13 * sin(q3);
h23 = J1 + J13 * sin(q3);
h32 = h23;
h33 = J1;

H = [h11, 0 ,0 ;
    0 , h22, h23;
    0 , h32, h33];

c12_1 = J1 * sin(2 * (q1 + q2)) - J12 * sin(2 * q2) + 2 * J13 * cos(2 * q2 +q3);
c13_1 = J1 * sin(2 * (q2 + q3)) + 2 * J13 * cos(q2) * cos(q2 + q3);
c11_2 = (1/2) * (-J1 * sin(2 * (q2 + q3)) + J12 * sin(2 * q2) - 2 * J13 * cos(2 * q2 + q3));
c22_2 = 2 * J13 * cos(q3);
c23_2 = J13 * cos(q3);
c22_3 = -J13 * cos(q3)* dq2;%NEED TO CHECK IF THIS IS CORRECT
c11_3 = (-1/2) * (J1 * sin(2 * (q2 + q3)) + J13 * cos(q2) * cos(q2 + q3));

C = [0, c12_1 * dq1, c13_1 * dq3;
    c11_2 * dq1, 0 , (c22_2)* dq2 + (c23_2)*dq3;
    c11_3 * dq1, c22_3 * dq2, 0];

g = 9.81;

g21 = -g * (lc3 * m3 * sin(q2 + q3) + lc2 * m2 * cos(q2) + l2 * m3 * cos(q2));
g31 = -g * (lc3 * m3 * sin(q2 + q3));

G = [0;
    g21;
    g31];

%% Define the Jacobian
jac=[-sin(q1)*(l3*sin(q2 + q3) + l2*cos(q2)), cos(q1)*(l3*cos(q2 + q3) - l2*sin(q2)), l3*cos(q2 + q3)*cos(q1);
 cos(q1)*(l3*sin(q2 + q3) + l2*cos(q2)), sin(q1)*(l3*cos(q2 + q3) - l2*sin(q2)), l3*cos(q2 + q3)*sin(q1);
                                      0,         - l3*sin(q2 + q3) - l2*cos(q2),        -l3*sin(q2 + q3)];
                                  
%% Define the derivative of the jacobian
dJac=[- sin(q1)*(l3*cos(q2 + q3)*(dq2 + dq3) - l2*sin(q2)*dq2) - cos(q1)*(l2*cos(q2) + l3*sin(q2 + q3))*dq1,   sin(q1)*dq1*(l2*sin(q2) - l3*cos(q2 + q3)) - cos(q1)*(l3*sin(q2 + q3)*(dq2 + dq3) + l2*cos(q2)*dq2), - l3*sin(q1)*cos(q2 + q3)*dq1 - l3*cos(q1)*sin(q2 + q3)*(dq2 + dq3);
  cos(q1)*(l3*cos(q2 + q3)*(dq2 + dq3) - l2*sin(q2)*dq2) - sin(q1)*(l2*cos(q2) + l3*sin(q2 + q3))*dq1, - sin(q1)*(l3*sin(q2 + q3)*(dq2 + dq3) + l2*cos(q2)*dq2) - cos(q1)*(l2*sin(q2) - l3*cos(q2 + q3))*dq1,   l3*cos(q1)*cos(q2 + q3)*dq1 - l3*sin(q1)*sin(q2 + q3)*(dq2 + dq3);
                                                                                                                                                                        0,                                                                                    l2*sin(q2)*dq2 - l3*cos(q2 + q3)*(dq2 + dq3),                                                               -l3*cos(q2 + q3)*(dq2 + dq3)];

%% Define the task space matrices
%Check to make sure we haven't hit a singularity
if det(jac)<10e-4
    jac=previousJacIn;
    previousJacOut=previousJacIn;
else
    previousJacOut=jac;
end

Hp=inv(transpose(jac))*H*inv(jac);
Cp=inv(transpose(jac))*C*inv(jac)-Hp*dJac*inv(jac);
Gp=inv(transpose(jac))*G;

%% Equivalent Task Space Vectors
p=[cos(q1)*(l3*sin(q2 + q3) + l2*cos(q2));sin(q1)*(l3*sin(q2 + q3) + l2*cos(q2));l1 + l3*cos(q2 + q3) - l2*sin(q2)];
pd=[cos(qd1)*(l3*sin(qd2 + qd3) + l2*cos(qd2));sin(qd1)*(l3*sin(qd2 + qd3) + l2*cos(qd2));l1 + l3*cos(qd2 + qd3) - l2*sin(qd2)];

dp=jac*dq;
dpd=jac*dqd;

ddpd=jac*ddqd+dJac*dqd;

%% Define our parrellel Decomposition
pr=pd+pf;
dpr=dpd+dpf;
ddpr=ddpd+ddpf;
                                  
%% Function output
%Define the stiffness and damping matrix below for task space directions
Km=[500 0 0;0 500 0;0 0 500];
Dm=[50 0 0;0 50 0;0 0 50];
Hm=diag([20,20,20]);

u0=ddpr+inv(Hp)*(Dm*(dpr-dp)+Km*(pr-p));
jacT=transpose(jac);
torque=jacT*(Hp*u0+Cp*dp+Gp-f);

test=Hp;

== matlab function pumaModel/Controller/Task Space Impedance Measurements/TaskSpaceImpedance_withMeasurements ==
  data: q input; dq input; ddq input; qd input; dqd input; torque output; ddqd input; f input
function torque     = ImpedanceControllerTaskSpace_Lectures_NoForceMeasurements(q,dq,ddq,qd,dqd,ddqd,f)
%% Joint Space variables
q1 = q(1);
q2 = q(2);
q3 = q(3);

dq1 = dq(1);
dq2 = dq(2);
dq3 = dq(3);

qd1 = qd(1);
qd2 = qd(2);
qd3 = qd(3);

% dqd1 = dqd(1);
% dqd2 = dqd(2);
% dqd3 = dqd(3);

%% Manipulator Geometry
l1 = 0.6731;
l2 = 0.432;
l3 = 0.434;
lc2 = 0.216;
lc3 = 0.164;
m2 = 15.46;
m3 = 9.55;
J = 0.302;

J1 = m3 * lc3^2;
J12 = (m2 * lc2^2) + (m3 * l2^2);
J13 = l2 * lc3 * m3;


h11 = J + J1 * (sin(q2 + q3))^2 + J12 * (cos(q2))^2 + 2 * J13 * cos(q2) * sin(q2+q3);
h22 = J1 + J12 + 2 * J13 * sin(q3);
h23 = J1 + J13 * sin(q3);
h32 = h23;
h33 = J1;

H = [h11, 0 ,0 ;
    0 , h22, h23;
    0 , h32, h33];

c12_1 = J1 * sin(2 * (q1 + q2)) - J12 * sin(2 * q2) + 2 * J13 * cos(2 * q2 +q3);
c13_1 = J1 * sin(2 * (q2 + q3)) + 2 * J13 * cos(q2) * cos(q2 + q3);
c11_2 = (1/2) * (-J1 * sin(2 * (q2 + q3)) + J12 * sin(2 * q2) - 2 * J13 * cos(2 * q2 + q3));
c22_2 = 2 * J13 * cos(q3);
c23_2 = J13 * cos(q3);
c22_3 = -J13 * cos(q3)* dq2;%NEED TO CHECK IF THIS IS CORRECT
c11_3 = (-1/2) * (J1 * sin(2 * (q2 + q3)) + J13 * cos(q2) * cos(q2 + q3));

C = [0, c12_1 * dq1, c13_1 * dq3;
    c11_2 * dq1, 0 , (c22_2)* dq2 + (c23_2)*dq3;
    c11_3 * dq1, c22_3 * dq2, 0];

g = 9.81;

g21 = -g * (lc3 * m3 * sin(q2 + q3) + lc2 * m2 * cos(q2) + l2 * m3 * cos(q2));
g31 = -g * (lc3 * m3 * sin(q2 + q3));

G = [0;
    g21;
    g31];

%% Define the Jacobian
jac=[-sin(q1)*(l3*sin(q2 + q3) + l2*cos(q2)), cos(q1)*(l3*cos(q2 + q3) - l2*sin(q2)), l3*cos(q2 + q3)*cos(q1);
 cos(q1)*(l3*sin(q2 + q3) + l2*cos(q2)), sin(q1)*(l3*cos(q2 + q3) - l2*sin(q2)), l3*cos(q2 + q3)*sin(q1);
                                      0,         - l3*sin(q2 + q3) - l2*cos(q2),        -l3*sin(q2 + q3)];
                                  
%% Define the derivative of the jacobian
dJac=[- sin(q1)*(l3*cos(q2 + q3)*(dq2 + dq3) - l2*sin(q2)*dq2) - cos(q1)*(l2*cos(q2) + l3*sin(q2 + q3))*dq1,   sin(q1)*dq1*(l2*sin(q2) - l3*cos(q2 + q3)) - cos(q1)*(l3*sin(q2 + q3)*(dq2 + dq3) + l2*cos(q2)*dq2), - l3*sin(q1)*cos(q2 + q3)*dq1 - l3*cos(q1)*sin(q2 + q3)*(dq2 + dq3);
  cos(q1)*(l3*cos(q2 + q3)*(dq2 + dq3) - l2*sin(q2)*dq2) - sin(q1)*(l2*cos(q2) + l3*sin(q2 + q3))*dq1, - sin(q1)*(l3*sin(q2 + q3)*(dq2 + dq3) + l2*cos(q2)*dq2) - cos(q1)*(l2*sin(q2) - l3*cos(q2 + q3))*dq1,   l3*cos(q1)*cos(q2 + q3)*dq1 - l3*sin(q1)*sin(q2 + q3)*(dq2 + dq3);
                                                                                                                                                                        0,                                                                                    l2*sin(q2)*dq2 - l3*cos(q2 + q3)*(dq2 + dq3),                                                               -l3*cos(q2 + q3)*(dq2 + dq3)];

%% Define the task space matrices
Hp=inv(transpose(jac))*H*inv(jac);
Cp=inv(transpose(jac))*C*inv(jac)-Hp*dJac*inv(jac);
Gp=inv(transpose(jac))*G;

%% Equivalent Task Space Vectors
p=[cos(q1)*(l3*sin(q2 + q3) + l2*cos(q2));sin(q1)*(l3*sin(q2 + q3) + l2*cos(q2));l1 + l3*cos(q2 + q3) - l2*sin(q2)];
pd=[cos(qd1)*(l3*sin(qd2 + qd3) + l2*cos(qd2));sin(qd1)*(l3*sin(qd2 + qd3) + l2*cos(qd2));l1 + l3*cos(qd2 + qd3) - l2*sin(qd2)];

dp=jac*dq;
dpd=jac*dqd;

% ddp=jac*ddq+dJac*dq;
ddpd=jac*ddqd+dJac*dqd;

                                  

%% Function output
%Define the stiffness and damping matrix below for task space directions
Km=[100 0 0;0 100 0;0 0 100];
Dm=[50 0 0;0 50 0;0 0 50];
Hm=diag([2 2 2]);

jacT=transpose(jac);
u0=ddpd+inv(Hm)*(Dm*(dpd-dp)+Km*(pd-p)+f);
torque=jacT*(Hp*u0+Cp*dp+Gp-f);

== matlab function pumaModel/Controller/Sliding Robust Control/SlidingRobustControl ==
  data: q input; dq input; qd input; dqd input; u output; ddqd input; dPhi input; phi input; S output
function [u,S]  = ImpedanceControllerTaskSpace(q,dq,qd,dqd,ddqd,dPhi,phi)
%% Unpackage the incoming reference/measured states
q1 = q(1);
q2 = q(2);
q3 = q(3);

qd1 = qd(1);
qd2 = qd(2);
qd3 = qd(3);

dq1 = dq(1);
dq2 = dq(2);
dq3 = dq(3);

dqd1 = dqd(1);
dqd2 = dqd(2);
dqd3 = dqd(3);

ddqd1=ddqd(1);
ddqd2=ddqd(2);
ddqd3=ddqd(3);

%% Define all the matrices of the manipulator
l1 = 0.6731;
l2 = 0.432;
l3 = 0.434;
lc2 = 0.216;
lc3 = 0.164;
m2 = 15.46;
m3 = 9.55;
J = 0.302;

% Inertia Matrix Parameters

J1 = m3 * lc3^2;
J12 = (m2 * lc2^2) + (m3 * l2^2);
J13 = l2 * lc3 * m3;


h11 = J + J1 * (sin(q2 + q3))^2 + J12 * (cos(q2))^2 + 2 * J13 * cos(q2) * sin(q2+q3);
h22 = J1 + J12 + 2 * J13 * sin(q3);
h23 = J1 + J13 * sin(q3);
h32 = h23;
h33 = J1;

H = [h11, 0 ,0 ;
    0 , h22, h23;
    0 , h32, h33];

% Coriolis Matrix Parameters

c12_1 = J1 * sin(2 * (q1 + q2)) - J12 * sin(2 * q2) + 2 * J13 * cos(2 * q2 +q3);
c13_1 = J1 * sin(2 * (q2 + q3)) + 2 * J13 * cos(q2) * cos(q2 + q3);
c11_2 = (1/2) * (-J1 * sin(2 * (q2 + q3)) + J12 * sin(2 * q2) - 2 * J13 * cos(2 * q2 + q3));
c22_2 = 2 * J13 * cos(q3);
c23_2 = J13 * cos(q3);
c22_3 = -J13 * cos(q3)* dq2;%NEED TO CHECK IF THIS IS CORRECT
c11_3 = (-1/2) * (J1 * sin(2 * (q2 + q3)) + J13 * cos(q2) * cos(q2 + q3));

C = [0, c12_1 * dq1, c13_1 * dq3;
    c11_2 * dq1, 0 , (c22_2)* dq2 + (c23_2)*dq3;
    c11_3 * dq1, c22_3 * dq2, 0];

% Vector of Potential Forces Parameters

g = 9.81;

g21 = -g * (lc3 * m3 * sin(q2 + q3) + lc2 * m2 * cos(q2) + l2 * m3 * cos(q2));
g31 = -g * (lc3 * m3 * sin(q2 + q3));

G = [0;
    g21;
    g31];

%% Sliding Mode Control Stuff
%Define all our own variables
qError=q-qd;
dqError=dq-dqd;

%Define sliding surface
lambda=50*eye(3);
S=dqError+lambda*qError;

%Define upperbound on expected system disturbances
% F=[662;932;4182];
F=[254;341;1800];

%Define neta, Used to avoid dividing by zero
neta=[1;1;1];

%Define Robust Term
K=F+neta-dPhi;
% K=F+neta;
robustTerm=K.*min(max(S./phi, -1), 1);%This is the saturation expression here

%Define fHat
fHat=inv(H)*(-G-C*dq);

%Define our complete control law
u=H*(-fHat+ddqd-lambda*dqError)-robustTerm;

== matlab function pumaModel/PUMA560/Manipulator Dynamic/MATLAB Function ==
  data: tau input; tau_e input; q input; ddq output; dq input
function ddq = DynamicModel( tau, tau_e, q, dq)
%%%%%
% 3-DOF Puma-560 Dynamic Model Function
% H(q)* ddq + C(q) * dq + G = tau + tau_e
% q is 3*1 vector of joint variables (radian)
% H(q) is the inertia matrix
% C(q) is the matrix of Coriolis and centrifugal forces
% G(q) is  the vector of potential forces Parameters
% tau is control torque 
% tau_e is the external torque due to the interaction with the environment
%%%%%

%% Joint Space variables

q1 = q(1);
q2 = q(2);
q3 = q(3);

dq1 = dq(1);
dq2 = dq(2);
dq3 = dq(3);

%% general physical parameters

l1 = 0.6731;
l2 = 0.432;
l3 = 0.434;
lc2 = 0.216;
lc3 = 0.164;
m2 = 15.46;
m3 = 9.55;
J = 0.302;

%% Inertia Matrix Parameters

J1 = m3 * lc3^2;
J12 = (m2 * lc2^2) + (m3 * l2^2);
J13 = l2 * lc3 * m3;


h11 = J + J1 * (sin(q2 + q3))^2 + J12 * (cos(q2))^2 + 2 * J13 * cos(q2) * sin(q2+q3);
h22 = J1 + J12 + 2 * J13 * sin(q3);
h23 = J1 + J13 * sin(q3);
h32 = h23;
h33 = J1;

H = [h11, 0 ,0 ;
    0 , h22, h23;
    0 , h32, h33];

%% Coriolis Matrix Parameters

c12_1 = J1 * sin(2 * (q1 + q2)) - J12 * sin(2 * q2) + 2 * J13 * cos(2 * q2 +q3);
c13_1 = J1 * sin(2 * (q2 + q3)) + 2 * J13 * cos(q2) * cos(q2 + q3);
c11_2 = (1/2) * (-J1 * sin(2 * (q2 + q3)) + J12 * sin(2 * q2) - 2 * J13 * cos(2 * q2 + q3));
c22_2 = 2 * J13 * cos(q3);
c23_2 = J13 * cos(q3);
c22_3 = -J13 * cos(q3) * dq2;
c11_3 = (-1/2) * (J1 * sin(2 * (q2 + q3)) + J13 * cos(q2) * cos(q2 + q3));

C = [0, c12_1 * dq1, c13_1 * dq3;
    c11_2 * dq1, 0 , ((c22_2))* dq2 + ((c23_2))*dq3;
    c11_3 * dq1, c22_3 * dq2, 0];

%% Vector of Potential Forces Parameters

g = 9.81;

g21 = -g * (lc3 * m3 * sin(q2 + q3) + lc2 * m2 * cos(q2) + l2 * m3 * cos(q2));
g31 = -g * (lc3 * m3 * sin(q2 + q3));

G = [0;
    g21;
    g31];

%% Function output

ddq = inv(H)*(tau + tau_e - C * dq - G);
